simulink model "sampleModel1595"  (R2023a)
settings: Solver=VariableStepAuto  StartTime=0.0  StopTime=10.0  RelTol=1e-3
libraries: simulink x3, hdlsllib x3
settings Model: Creator=user1  LastModifiedBy=user1

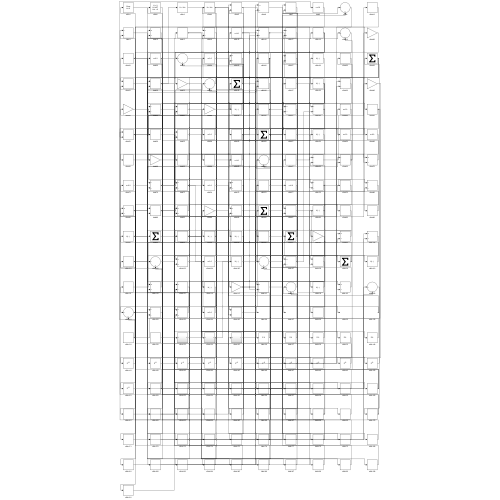
[thumbnail: Simulink's stored preview of the top-level diagram]
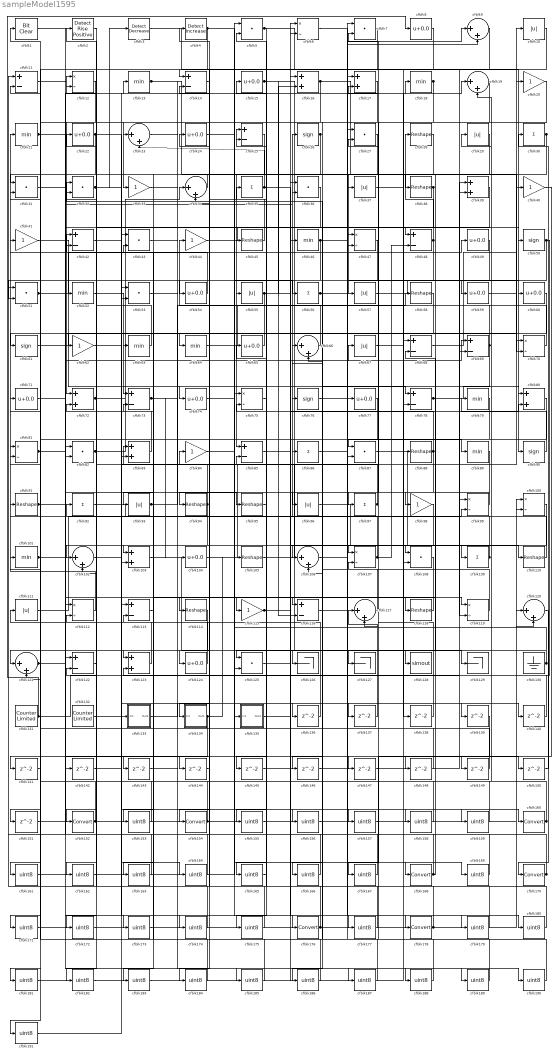
== system sampleModel1595 ==
  cfblk1 : simulink/Logic and Bit Operations/Bit Clear  iBit=0
      settings: LibrarySourceBlock=|
      | hdlsllib/Logic and Bit
      | Operations/Bit Clear
  cfblk{10,29,37,55,57,67,93,96,111} (9 alike) : Abs  SaturateOnIntegerOverflow=off
  cfblk{6,12,47,70,75,81,99..100,107,112,119} (11 alike) : Product  Inputs=*/  RndMeth=Zero  SaturateOnIntegerOverflow=on
  cfblk{13,18,21,46,52,63..64,79,89,101} (10 alike) : MinMax
  cfblk{9,19,23,34,66,102,106,117,120..121} (10 alike) : Sum  Inputs=|++
  cfblk{16..17,39,72,80,83,103,123} (8 alike) : Sum
  cfblk{8,15,22,24,49,54,59..60,65,71,74,77,104,124} (14 alike) : Bias  Bias=0.0  SaturateOnIntegerOverflow=off
  cfblk{28,38,45,58,88,91,94..95,105,110,114,118} (12 alike) : Reshape
  cfblk{5,7,27,31..32,36,43,51,53,82,87,108,125} (13 alike) : DotProduct  OutDataTypeStr=Inherit: Inherit via internal rule
  cfblk{30,35,56,86,92,97,109} (7 alike) : Sum  Inputs=+
  cfblk{11,14,25,42,48,68..69,73,78,85,113,116,122} (13 alike) : Sum  Inputs=+-
  cfblk{20,33,40..41,44,62,84,98,115} (9 alike) : Gain
  cfblk126 : Terminator
  cfblk127 : Terminator
  cfblk128 : ToWorkspace  VariableName=simout  SaveFormat=Timeseries  SampleTime=-1
  cfblk129 : Terminator
  cfblk130 : Ground
  cfblk131 : hdlsllib/Sources/Counter Limited  uplimit=7  tsamp=-1
  cfblk132 : hdlsllib/Sources/Counter Limited  uplimit=7  tsamp=-1
  cfblk133 : Subsystem
      settings: LibrarySourceBlock=|
      | hdlsllib/Ports &
      | Subsystems/Subsystem
  cfblk134 : Subsystem
      settings: LibrarySourceBlock=|
      | hdlsllib/Ports &
      | Subsystems/Subsystem
  cfblk135 : Subsystem
      settings: LibrarySourceBlock=|
      | hdlsllib/Ports &
      | Subsystems/Subsystem
  cfblk{136..151} (16 alike) : Delay  SampleTime=1
  cfblk{152,154,160,168,170,176,178} (7 alike) : DataTypeConversion  SaturateOnIntegerOverflow=off  RndMeth=Floor
  cfblk{153,155..159,161..167,169,171..175,177,179..191} (33 alike) : DataTypeConversion  OutDataTypeStr=uint8  SaturateOnIntegerOverflow=off  RndMeth=Floor
  cfblk2 : hdlsllib/Logic and Bit Operations/Detect Rise Positive  vinit=0  OutDataTypeStr=boolean
  cfblk{26,50,61,76,90} (5 alike) : Signum
  cfblk3 : simulink/Logic and Bit Operations/Detect Decrease  vinit=0.0  OutDataTypeStr=boolean
      settings: LibrarySourceBlock=|
      | hdlsllib/Logic and Bit
      | Operations/Detect
      | Decrease
  cfblk4 : simulink/Logic and Bit Operations/Detect Increase  vinit=0.0  OutDataTypeStr=boolean
      settings: LibrarySourceBlock=|
      | hdlsllib/Logic and Bit
      | Operations/Detect
      | Increase
  wires:
  cfblk54/1 -> cfblk21/1
  cfblk48/1 -> cfblk28/1, cfblk125/2, cfblk66/2
  cfblk112/1 -> cfblk41/1
  cfblk77/1 -> cfblk123/1
  cfblk131/1 -> cfblk8/1, cfblk39/2
  cfblk34/1 -> cfblk31/1
  cfblk82/1 -> cfblk34/1, cfblk85/2
  cfblk135/1(Out1) -> cfblk160/1
  cfblk72/1 -> cfblk74/1, cfblk18/1
  cfblk66/1 -> cfblk44/1
  cfblk97/1 -> cfblk83/1, cfblk12/2
  cfblk13/1 -> cfblk57/1, cfblk47/1
  cfblk12/1 -> cfblk72/1
  cfblk32/1 -> cfblk3/1, cfblk174/1
  cfblk14/1 -> cfblk64/1
  cfblk1/1 -> cfblk48/1
  cfblk119/1 -> cfblk91/1
  cfblk120/1 -> cfblk170/1
  cfblk96/1 -> cfblk109/1
  cfblk15/1 -> cfblk127/1, cfblk116/2
  cfblk100/1 -> cfblk154/1
  cfblk22/1 -> cfblk42/2, cfblk136/1
  cfblk87/1 -> cfblk110/1
  cfblk52/1 -> cfblk73/1
  cfblk99/1 -> cfblk98/1
  cfblk46/1 -> cfblk77/1, cfblk51/2
  cfblk124/1 -> cfblk71/1
  cfblk89/1 -> cfblk128/1
  cfblk21/1 -> cfblk116/1, cfblk70/2
  cfblk121/1 -> cfblk67/1, cfblk143/1
  cfblk38/1 -> cfblk83/2, cfblk52/1, cfblk182/1
  cfblk107/1 -> cfblk1/1, cfblk48/2
  cfblk111/1 -> cfblk26/1
  cfblk2/1 -> cfblk152/1
  cfblk9/1 -> cfblk14/1
  cfblk4/1 -> cfblk56/1, cfblk38/1, cfblk191/1
  cfblk25/1 -> cfblk94/1
  cfblk65/1 -> cfblk61/1
  cfblk39/1 -> cfblk85/1
  cfblk83/1 -> cfblk42/1
  cfblk29/1 -> cfblk108/1
  cfblk20/1 -> cfblk33/1
  cfblk3/1 -> cfblk90/1
  cfblk123/1 -> cfblk81/1
  cfblk110/1 -> cfblk14/2
  cfblk50/1 -> cfblk117/1, cfblk103/2
  cfblk61/1 -> cfblk63/1
  cfblk63/1 -> cfblk12/1
  cfblk93/1 -> cfblk58/1, cfblk150/1, cfblk185/1
  cfblk115/1 -> cfblk80/2, cfblk179/1
  cfblk57/1 -> cfblk60/1
  cfblk103/1 -> cfblk126/1
  cfblk69/1 -> cfblk29/1, cfblk25/2, cfblk166/1
  cfblk30/1 -> cfblk55/1, cfblk121/2, cfblk96/1
  cfblk18/1 -> cfblk23/1, cfblk124/1, cfblk141/1
  cfblk44/1 -> cfblk50/1
  cfblk78/1 -> cfblk80/1, cfblk118/1
  cfblk85/1 -> cfblk119/1
  cfblk45/1 -> cfblk4/1
  cfblk101/1 -> cfblk69/1, cfblk190/1
  cfblk28/1 -> cfblk82/2
  cfblk19/1 -> cfblk97/1
  cfblk16/1 -> cfblk70/1, cfblk102/2
  cfblk8/1 -> cfblk54/1
  cfblk134/1(Out1) -> cfblk105/1, cfblk151/1
  cfblk104/1 -> cfblk40/1
  cfblk70/1 -> cfblk35/1
  cfblk130/1 -> cfblk125/1, cfblk107/2
  cfblk10/1 -> cfblk119/2
  cfblk64/1 -> cfblk46/1
  cfblk92/1 -> cfblk99/2
  cfblk59/1 -> cfblk10/1
  cfblk117/1 -> cfblk32/1
  cfblk79/1 -> cfblk87/1
  cfblk73/1 -> cfblk104/1, cfblk177/1
  cfblk27/1 -> cfblk114/1
  cfblk35/1 -> cfblk23/2, cfblk147/1
  cfblk74/1 -> cfblk129/1
  cfblk24/1 -> cfblk176/1
  cfblk86/1 -> cfblk178/1
  cfblk116/1 -> cfblk9/1
  cfblk51/1 -> cfblk49/1, cfblk16/1
  cfblk68/1 -> cfblk20/1
  cfblk81/1 -> cfblk13/1, cfblk36/2
  cfblk88/1 -> cfblk15/1, cfblk134/1(In1)
  cfblk56/1 -> cfblk59/1, cfblk9/2, cfblk108/2
  cfblk105/1 -> cfblk39/1
  cfblk55/1 -> cfblk93/1, cfblk107/1, cfblk16/2
  cfblk109/1 -> cfblk25/1, cfblk102/1
  cfblk94/1 -> cfblk73/2, cfblk172/1
  cfblk118/1 -> cfblk115/1
  cfblk91/1 -> cfblk112/1, cfblk95/1
  cfblk41/1 -> cfblk78/1
  cfblk84/1 -> cfblk168/1
  cfblk67/1 -> cfblk19/1
  cfblk76/1 -> cfblk89/1
  cfblk47/1 -> cfblk121/1
  cfblk5/1 -> cfblk45/1, cfblk78/2
  cfblk26/1 -> cfblk62/1, cfblk103/1, cfblk145/1
  cfblk98/1 -> cfblk106/1
  cfblk90/1 -> cfblk79/1
  cfblk136/1 -> cfblk82/1
  cfblk133/1(Out1) -> cfblk137/1
  cfblk137/1 -> cfblk5/1
  cfblk37/1 -> cfblk138/1
  cfblk138/1 -> cfblk7/1
  cfblk33/1 -> cfblk139/1
  cfblk23/1 -> cfblk140/1
  cfblk140/1 -> cfblk123/2
  cfblk141/1 -> cfblk81/2
  cfblk71/1 -> cfblk142/1
  cfblk62/1 -> cfblk144/1
  cfblk144/1 -> cfblk34/2
  cfblk145/1 -> cfblk69/2
  cfblk49/1 -> cfblk146/1
  cfblk146/1 -> cfblk99/1
  cfblk147/1 -> cfblk117/2
  cfblk102/1 -> cfblk148/1
  cfblk148/1 -> cfblk112/2
  cfblk40/1 -> cfblk149/1
  cfblk149/1 -> cfblk31/2
  cfblk150/1 -> cfblk30/1
  cfblk151/1 -> cfblk88/1
  cfblk152/1 -> cfblk47/2, cfblk111/1
  cfblk36/1 -> cfblk153/1
  cfblk153/1 -> cfblk2/1
  cfblk154/1 -> cfblk87/2, cfblk72/2
  cfblk58/1 -> cfblk155/1
  cfblk155/1 -> cfblk100/1
  cfblk132/1 -> cfblk156/1
  cfblk156/1 -> cfblk100/2
  cfblk43/1 -> cfblk157/1
  cfblk157/1 -> cfblk7/2
  cfblk106/1 -> cfblk158/1
  cfblk158/1 -> cfblk43/1
  cfblk142/1 -> cfblk159/1
  cfblk159/1 -> cfblk43/2
  cfblk160/1 -> cfblk19/2, cfblk36/1, cfblk92/1
  cfblk114/1 -> cfblk161/1
  cfblk161/1 -> cfblk135/1(In1)
  cfblk122/1 -> cfblk162/1
  cfblk162/1 -> cfblk133/1(In1)
  cfblk108/1 -> cfblk163/1
  cfblk163/1 -> cfblk122/1
  cfblk42/1 -> cfblk164/1
  cfblk164/1 -> cfblk122/2
  cfblk75/1 -> cfblk165/1
  cfblk165/1 -> cfblk5/2
  cfblk166/1 -> cfblk75/1
  cfblk139/1 -> cfblk167/1
  cfblk167/1 -> cfblk75/2
  cfblk168/1 -> cfblk68/2, cfblk51/1
  cfblk125/1 -> cfblk169/1
  cfblk169/1 -> cfblk84/1
  cfblk170/1 -> cfblk66/1, cfblk22/1
  cfblk7/1 -> cfblk171/1
  cfblk171/1 -> cfblk120/1
  cfblk172/1 -> cfblk120/2
  cfblk11/1 -> cfblk173/1
  cfblk173/1 -> cfblk37/1
  cfblk174/1 -> cfblk11/1
  cfblk95/1 -> cfblk175/1
  cfblk175/1 -> cfblk11/2
  cfblk176/1 -> cfblk32/2, cfblk65/1
  cfblk177/1 -> cfblk24/1
  cfblk178/1 -> cfblk106/2, cfblk27/1
  cfblk179/1 -> cfblk86/1
  cfblk6/1 -> cfblk180/1
  cfblk180/1 -> cfblk27/2
  cfblk80/1 -> cfblk181/1
  cfblk181/1 -> cfblk6/1
  cfblk182/1 -> cfblk6/2
  cfblk113/1 -> cfblk183/1
  cfblk183/1 -> cfblk68/1
  cfblk60/1 -> cfblk184/1
  cfblk184/1 -> cfblk113/1
  cfblk185/1 -> cfblk113/2
  cfblk17/1 -> cfblk186/1
  cfblk186/1 -> cfblk101/1
  cfblk31/1 -> cfblk187/1
  cfblk187/1 -> cfblk17/1
  cfblk143/1 -> cfblk188/1
  cfblk188/1 -> cfblk17/2
  cfblk53/1 -> cfblk189/1
  cfblk189/1 -> cfblk76/1
  cfblk190/1 -> cfblk53/1
  cfblk191/1 -> cfblk53/2

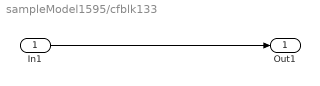
== system sampleModel1595/cfblk133 ==
  In1 : Inport
  Out1 : Outport
  wires:
  In1/1 -> Out1/1

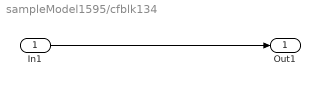
== system sampleModel1595/cfblk134 ==
  In1 : Inport
  Out1 : Outport
  wires:
  In1/1 -> Out1/1

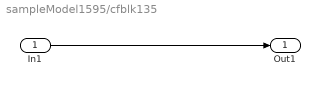
== system sampleModel1595/cfblk135 ==
  In1 : Inport
  Out1 : Outport
  wires:
  In1/1 -> Out1/1
